simulink model "sat_dist_sim"  (R2023b)
settings: Solver=VariableStepAuto  StartTime=0.0  StopTime=10.0  RelTol=1e-3
values from neighbouring files (symbols this model uses):
  A = [0.49 0.49 0.49 0.49 0.49 0.49 0.49 0.49 0.49 0.49 0.49 0.49 0.49 0.49]    [disturbances_report.m]    (also in sat_dist.m = [6*1e-2; 6*1e-2; 6*1e-2; 6*1e-2; 4*1e-2; 4*1e-2; 12*1e-2; 12)
  a = 1 / ( (2/r) - (v^2 / mu) )    [car2par.m]    (also in disturbances_report.m = 6851.22197053)
  A0 = eye(3)    [sat_dist.m]
  e = norm(ee)    [car2par.m]    (also in disturbances_report.m = 0.00183012221618)
  e3 = [1; 0; 0]    [sat_dist.m]
  epsilon = astroConstants(8)    [sat_dist.m]
  H0 = sqrt(g01^2+g11^2+h11^2)*1e-9    [disturbances_report.m]    (also in sat_dist.m)
  I = diag([I1 I2 I3])    [sat_dist.m]
  i_matrix = [1 0 0;0 cos(i) sin(i); 0 -sin(i) cos(i)]    [sat_dist.m]
  Iinv = I\eye(3)    [sat_dist.m]
  incl = deg2rad(11.5)    [disturbances_report.m]    (also in sat_dist.m)
  jb = [0.01; 0.05; 0.01]    [disturbances_report.m]    (also in sat_dist.m)
  mu = 3.986 * 10^5    (= 398600)    [car2par.m]    (also in sat_dist.m = astroConstants(13))
  n = sqrt(mu/a^3)    [sat_dist.m]
  N = [1 0 0]'    [car2par.m]    (also in disturbances_report.m = [0 1 0; 0 -1 0; sqrt(2)/2 0 sqrt(2)/2; -sqrt(2)/2 0 sqrt(2)/; sat_dist.m = [1 0 0; 0 1 0; -1 0 0; 0 -1 0; 0 0 1; 0 0 -1; 1 0 0; -1 0 0;)
  ns = 2*pi / Ts    (= 1.99098639111e-07)    [sat_dist.m]
  omega0 = zeros(3,1)    [disturbances_report.m]    (also in sat_dist.m = [0; 0; n])
  omegaE = deg2rad(15)/3600    [disturbances_report.m]    (also in sat_dist.m)
  P = astroConstants(31)/(astroConstants(5)*10^3)    [disturbances_report.m]    (also in sat_dist.m = Fe/c)
  rf = 1e-2*[10 0 0; 0 10 0; -10 0 0; 0 -10 0; 0 0 15; 0 0 -15; 0 0 45; 0 0 45; 0 0 -45; 0 0 -45]    [sat_dist.m]
  rhod = 0.1*ones(10,1)    [sat_dist.m]
  rhos = 0.5*ones(10,1)    [sat_dist.m]
  rhos_ = ones(10,1)-rhos    [sat_dist.m]
  rs = -rr    [disturbances_report.m]    (also in sat_dist.m = astroConstants(2))
  Rt = astroConstants(23)    [disturbances_report.m]    (also in sat_dist.m)
  s0 = zeros(3,1)    [disturbances_report.m]    (also in sat_dist.m)
undefined symbols (not defined in the file or in its folder): phi0, psi0, theta0
libraries: matrix_library x13
settings Model: Creator=marcellopareschi  LastModifiedBy=marcellopareschi

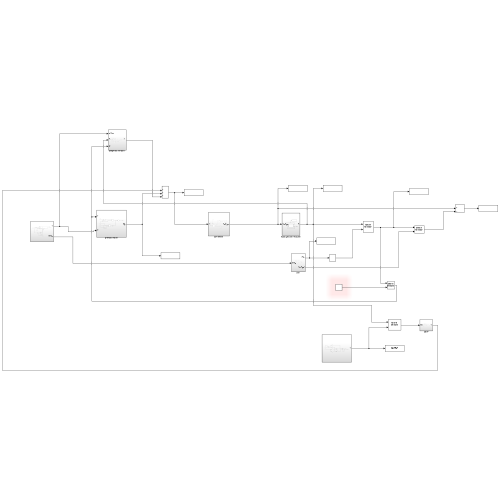
[thumbnail: Simulink's stored preview of the top-level diagram]
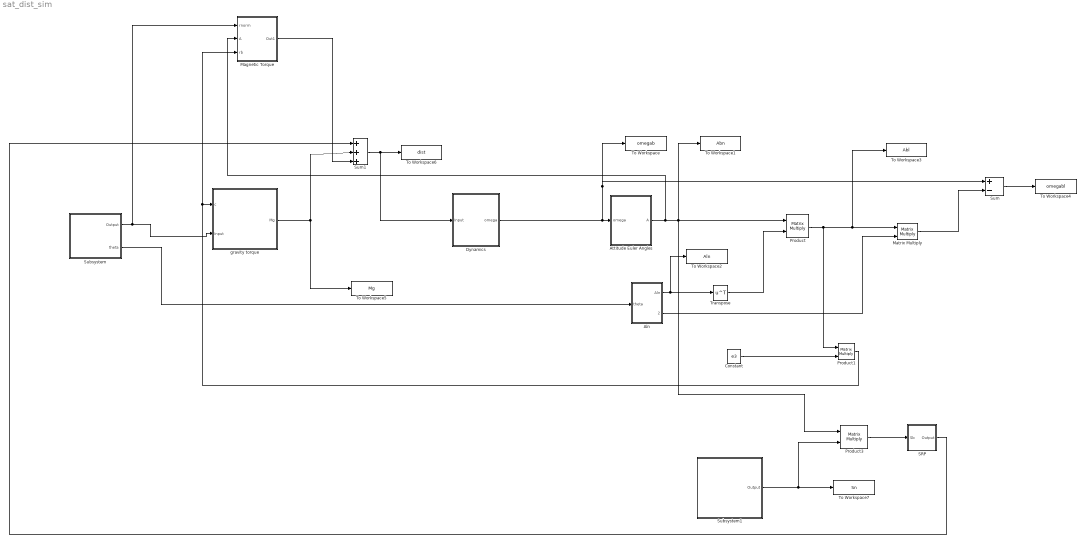
== system sat_dist_sim ==
  Aln : Subsystem
  Attitude Euler Angles : Subsystem
  Constant : Constant  Value=e3
  Dynamics : Subsystem
  "Magnetic Torque " : Subsystem
  Matrix Multiply : Product  Multiplication=Matrix(*)
  Product : Product  Multiplication=Matrix(*)
  Product1 : Product  Multiplication=Matrix(*)
  Product3 : Product  Multiplication=Matrix(*)
  SRP : Subsystem
  Subsystem : Subsystem
  Subsystem1 : Subsystem
  Sum : Sum  Inputs=|+-
  Sum1 : Sum  Inputs=|+++
  To Workspace : ToWorkspace  VariableName=omegab  SampleTime=-1
  To Workspace1 : ToWorkspace  VariableName=Abn  SampleTime=-1
  To Workspace2 : ToWorkspace  VariableName=Aln  SampleTime=-1
  To Workspace3 : ToWorkspace  VariableName=Abl  SampleTime=-1
  To Workspace4 : ToWorkspace  VariableName=omegabl  SampleTime=-1
  To Workspace5 : ToWorkspace  VariableName=Mg  SampleTime=-1
  To Workspace6 : ToWorkspace  VariableName=dist  SampleTime=-1
  To Workspace7 : ToWorkspace  VariableName=Sn  SampleTime=-1
  Transpose : Math  Operator=transpose
  gravity torque : Subsystem
  wires:
  Sum/1 -> To Workspace4/1
  Attitude Euler Angles/1(A) -> "Magnetic Torque "/2(A), Product3/1, To Workspace1/1, Product/1
  Product/1 -> To Workspace3/1, Matrix Multiply/1, Product1/1
  Aln/2(omegal) -> Matrix Multiply/2
  Transpose/1 -> Product/2
  Subsystem/2(theta) -> Aln/1(theta)
  Subsystem/1(Output) -> "Magnetic Torque "/1(rnorm), gravity torque/2(Input)
  Dynamics/1(omega) -> To Workspace/1, Sum/1, Attitude Euler Angles/1(omega)
  Aln/1(Aln) -> To Workspace2/1, Transpose/1
  Product3/1 -> SRP/1(Sb)
  Constant/1 -> Product1/2
  Product1/1 -> "Magnetic Torque "/3(rb), gravity torque/1(c)
  gravity torque/1(Mg) -> Sum1/2, To Workspace5/1
  Matrix Multiply/1 -> Sum/2
  SRP/1(Output) -> Sum1/1
  Subsystem1/1(Output) -> To Workspace7/1, Product3/2
  Sum1/1 -> Dynamics/1(Input), To Workspace6/1
  "Magnetic Torque "/1(Out1) -> Sum1/3

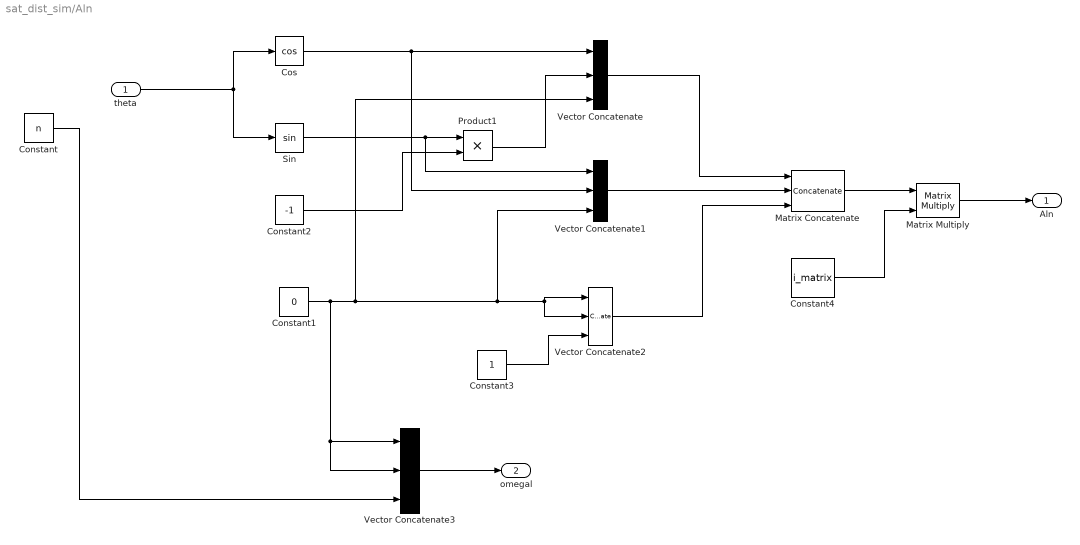
== system sat_dist_sim/Aln ==
  theta : Inport
  Constant : Constant  Value=n
  Constant1 : Constant  Value=0
  Constant2 : Constant  Value=-1
  Constant3 : Constant
  Constant4 : Constant  Value=i_matrix
  Cos : Trigonometry  Operator=cos
  Matrix Concatenate : Concatenate  NumInputs=3  Mode=Multidimensional array  ConcatenateDimension=2
  Matrix Multiply : Product  Multiplication=Matrix(*)
  Product1 : Product
  Sin : Trigonometry
  Vector Concatenate{,1..3} (4 alike) : Concatenate  NumInputs=3
  Aln : Outport
  omegal : Outport  Port=2
  wires:
  Constant/1 -> Vector Concatenate3/3
  Cos/1 -> Vector Concatenate1/2, Vector Concatenate/1
  Sin/1 -> Vector Concatenate1/1, Product1/1
  Constant2/1 -> Product1/2
  Product1/1 -> Vector Concatenate/2
  Constant1/1 -> Vector Concatenate3/1, Vector Concatenate3/2, Vector Concatenate/3, Vector Concatenate2/2, Vector Concatenate2/1, Vector Concatenate1/3
  Constant3/1 -> Vector Concatenate2/3
  Vector Concatenate/1 -> Matrix Concatenate/1
  Vector Concatenate1/1 -> Matrix Concatenate/2
  Vector Concatenate2/1 -> Matrix Concatenate/3
  Vector Concatenate3/1 -> omegal/1
  theta/1 -> Sin/1, Cos/1
  Matrix Concatenate/1 -> Matrix Multiply/1
  Constant4/1 -> Matrix Multiply/2
  Matrix Multiply/1 -> Aln/1

== system sat_dist_sim/Attitude Euler Angles ==
  omega : Inport
  Subsystem1 : Subsystem
  To Workspace : ToWorkspace  VariableName=angles  SampleTime=-1
  A : Outport
  wires:
  omega/1 -> Subsystem1/1(In1)
  Subsystem1/1(Angles) -> To Workspace/1, Subsystem1/2(Input)
  Subsystem1/2(A) -> Subsystem1/3(Input1), A/1

== system sat_dist_sim/Dynamics ==
  Input : Inport
  Constant : Constant  Value=I
  Constant1 : Constant  Value=Iinv
  Cross Product : matrix_library/Cross Product
  Integrator : Integrator  InitialCondition=omega0
  Product : Product  Multiplication=Matrix(*)
  Product1 : Product  Multiplication=Matrix(*)
  Scope : Scope
  Sum : Sum  Inputs=|++
  omega : Outport
  wires:
  Constant/1 -> Product/1
  Product1/1 -> Integrator/1
  Integrator/1 -> omega/1, Scope/1, Product/2, Cross Product/2
  Product/1 -> Cross Product/1
  Constant1/1 -> Product1/1
  Cross Product/1 -> Sum/1
  Sum/1 -> Product1/2
  Input/1 -> Sum/2

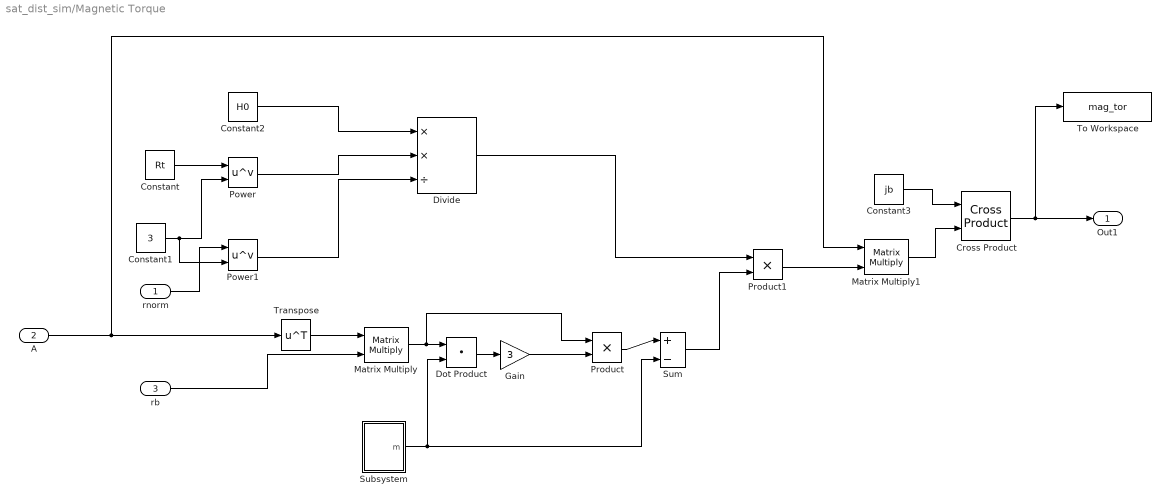
== system sat_dist_sim/Magnetic Torque  ==
  rnorm : Inport
  A : Inport  Port=2
  rb : Inport  Port=3
  Constant : Constant  Value=Rt
  Constant1 : Constant  Value=3
  Constant2 : Constant  Value=H0
  Constant3 : Constant  Value=jb
  Cross Product : matrix_library/Cross Product
  Divide : Product  Inputs=**/
  Dot Product : DotProduct  OutDataTypeStr=Inherit: Inherit via internal rule
  Gain : Gain  Gain=3
  Matrix Multiply : Product  Multiplication=Matrix(*)
  Matrix Multiply1 : Product  Multiplication=Matrix(*)
  Power : Math  Operator=pow
  Power1 : Math  Operator=pow
  Product : Product
  Product1 : Product
  Subsystem : Subsystem
  Sum : Sum  Inputs=|+-
  To Workspace : ToWorkspace  VariableName=mag_tor  SampleTime=-1
  Transpose : Math  Operator=transpose
  Out1 : Outport
  wires:
  A/1 -> Matrix Multiply1/1, Transpose/1
  Transpose/1 -> Matrix Multiply/1
  rb/1 -> Matrix Multiply/2
  Matrix Multiply/1 -> Product/1, Dot Product/1
  Subsystem/1(m) -> Sum/2, Dot Product/2
  Dot Product/1 -> Gain/1
  Gain/1 -> Product/2
  Product/1 -> Sum/1
  Constant/1 -> Power/1
  Constant1/1 -> Power1/2, Power/2
  rnorm/1 -> Power1/1
  Constant2/1 -> Divide/1
  Power/1 -> Divide/2
  Power1/1 -> Divide/3
  Divide/1 -> Product1/1
  Sum/1 -> Product1/2
  Product1/1 -> Matrix Multiply1/2
  Constant3/1 -> Cross Product/1
  Matrix Multiply1/1 -> Cross Product/2
  Cross Product/1 -> To Workspace/1, Out1/1

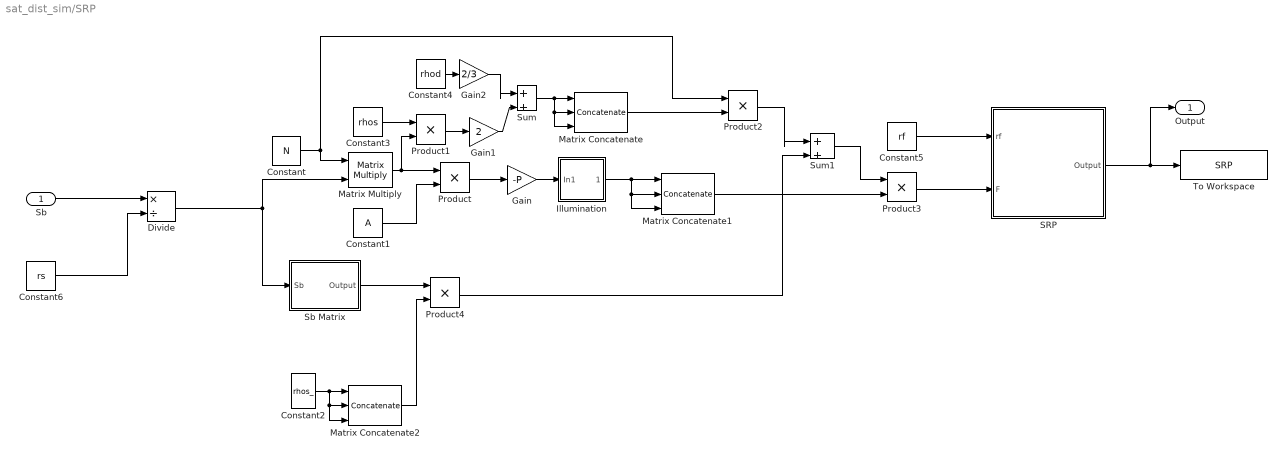
== system sat_dist_sim/SRP ==
  Sb : Inport
  Constant : Constant  Value=N
  Constant1 : Constant  Value=A
  Constant2 : Constant  Value=rhos_
  Constant3 : Constant  Value=rhos
  Constant4 : Constant  Value=rhod
  Constant5 : Constant  Value=rf
  Constant6 : Constant  Value=rs
  Divide : Product  Inputs=*/
  Gain : Gain  Gain=-P
  Gain1 : Gain  Gain=2
  Gain2 : Gain  Gain=2/3
  Illumination : Subsystem
  Matrix Concatenate : Concatenate  NumInputs=3  Mode=Multidimensional array  ConcatenateDimension=2
  Matrix Concatenate1 : Concatenate  NumInputs=3  Mode=Multidimensional array  ConcatenateDimension=2
  Matrix Concatenate2 : Concatenate  NumInputs=3  Mode=Multidimensional array  ConcatenateDimension=2
  Matrix Multiply : Product  Multiplication=Matrix(*)
  Product{,1..4} (5 alike) : Product
  SRP : Subsystem
  Sb Matrix : Subsystem
  Sum : Sum  Inputs=|++
  Sum1 : Sum  Inputs=|++
  To Workspace : ToWorkspace  VariableName=SRP  SampleTime=-1
  Output : Outport
  wires:
  Constant/1 -> Product2/1, Matrix Multiply/1
  Matrix Multiply/1 -> Product1/2, Product/1
  Constant1/1 -> Product/2
  Product/1 -> Gain/1
  Constant3/1 -> Product1/1
  Product1/1 -> Gain1/1
  Constant4/1 -> Gain2/1
  Gain2/1 -> Sum/1
  Gain1/1 -> Sum/2
  Sum/1 -> Matrix Concatenate/3, Matrix Concatenate/2, Matrix Concatenate/1
  Matrix Concatenate/1 -> Product2/2
  Gain/1 -> Illumination/1(In1)
  Product2/1 -> Sum1/1
  Matrix Concatenate1/1 -> Product3/2
  Sum1/1 -> Product3/1
  Constant5/1 -> SRP/1(rf)
  Product3/1 -> SRP/2(F)
  Constant2/1 -> Matrix Concatenate2/3, Matrix Concatenate2/2, Matrix Concatenate2/1
  Sb Matrix/1(Output) -> Product4/1
  Matrix Concatenate2/1 -> Product4/2
  Product4/1 -> Sum1/2
  Sb/1 -> Divide/1
  Constant6/1 -> Divide/2
  Divide/1 -> Sb Matrix/1(Sb), Matrix Multiply/2
  Illumination/1(Output) -> Matrix Concatenate1/3, Matrix Concatenate1/2, Matrix Concatenate1/1
  SRP/1(Output) -> To Workspace/1, Output/1

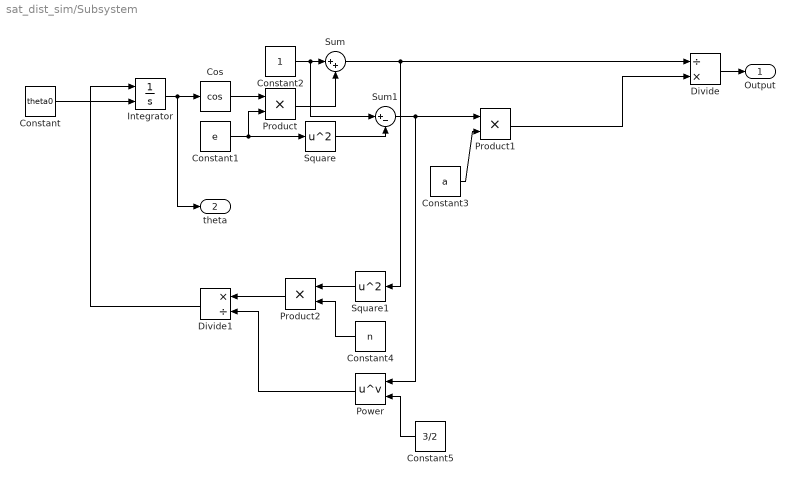
== system sat_dist_sim/Subsystem ==
  Constant : Constant  Value=theta0
  Constant1 : Constant  Value=e
  Constant2 : Constant
  Constant3 : Constant  Value=a
  Constant4 : Constant  Value=n
  Constant5 : Constant  Value=3/2
  Cos : Trigonometry  Operator=cos
  Divide : Product  Inputs=/*
  Divide1 : Product  Inputs=*/
  Integrator : Integrator  InitialConditionSource=external
  Power : Math  Operator=pow
  Product : Product
  Product1 : Product
  Product2 : Product
  Square : Math  Operator=square
  Square1 : Math  Operator=square
  Sum : Sum  Inputs=|++
  Sum1 : Sum  Inputs=|+-
  Output : Outport
  theta : Outport  Port=2
  wires:
  Constant/1 -> Integrator/2
  Integrator/1 -> theta/1, Cos/1
  Cos/1 -> Product/1
  Constant1/1 -> Square/1, Product/2
  Constant2/1 -> Sum1/1, Sum/1
  Product/1 -> Sum/2
  Square/1 -> Sum1/2
  Sum1/1 -> Power/1, Product1/1
  Constant3/1 -> Product1/2
  Product1/1 -> Divide/2
  Sum/1 -> Square1/1, Divide/1
  Square1/1 -> Product2/1
  Constant4/1 -> Product2/2
  Constant5/1 -> Power/2
  Product2/1 -> Divide1/1
  Power/1 -> Divide1/2
  Divide1/1 -> Integrator/1
  Divide/1 -> Output/1

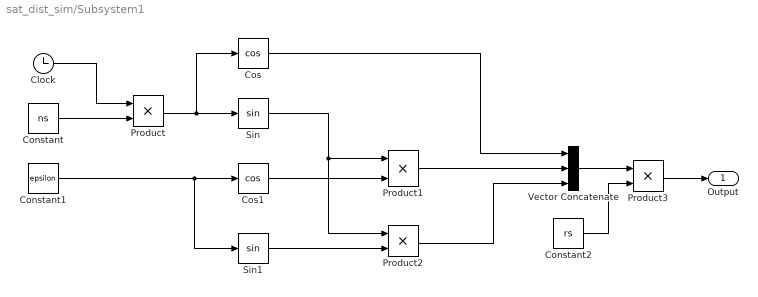
== system sat_dist_sim/Subsystem1 ==
  Clock : Clock
  Constant : Constant  Value=ns
  Constant1 : Constant  Value=epsilon
  Constant2 : Constant  Value=rs
  Cos : Trigonometry  Operator=cos
  Cos1 : Trigonometry  Operator=cos
  Product{,1..3} (4 alike) : Product
  Sin : Trigonometry
  Sin1 : Trigonometry
  Vector Concatenate : Concatenate  NumInputs=3
  Output : Outport
  wires:
  Constant/1 -> Product/2
  Clock/1 -> Product/1
  Product/1 -> Cos/1, Sin/1
  Constant1/1 -> Sin1/1, Cos1/1
  Sin/1 -> Product2/1, Product1/1
  Cos1/1 -> Product1/2
  Sin1/1 -> Product2/2
  Cos/1 -> Vector Concatenate/1
  Product1/1 -> Vector Concatenate/2
  Product2/1 -> Vector Concatenate/3
  Vector Concatenate/1 -> Product3/1
  Constant2/1 -> Product3/2
  Product3/1 -> Output/1

== system sat_dist_sim/gravity torque ==
  c : Inport
  Input : Inport  Port=2
  Constant : Constant  Value=mu
  Constant1 : Constant  Value=I
  Constant3 : Constant  Value=3
  Cross Product : matrix_library/Cross Product
  Divide : Product  Inputs=**/
  Gain : Gain  Gain=-1
  Matrix Multiply : Product  Multiplication=Matrix(*)
  Power : Math  Operator=pow
  Product : Product
  Mg : Outport
  wires:
  Constant1/1 -> Matrix Multiply/1
  c/1 -> Matrix Multiply/2, Cross Product/2
  Matrix Multiply/1 -> Cross Product/1
  Constant3/1 -> Power/2, Divide/2
  Power/1 -> Divide/3
  Constant/1 -> Divide/1
  Divide/1 -> Gain/1
  Gain/1 -> Product/2
  Cross Product/1 -> Product/1
  Product/1 -> Mg/1
  Input/1 -> Power/1

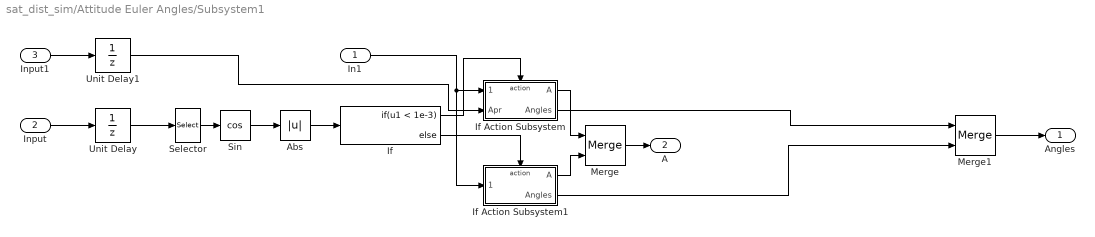
== system sat_dist_sim/Attitude Euler Angles/Subsystem1 ==
  In1 : Inport
  Input : Inport  Port=2
  Input1 : Inport  Port=3
  Abs : Abs  SaturateOnIntegerOverflow=off
  If : If  IfExpression=u1 < 1e-3
  If Action Subsystem : Subsystem  TreatAsAtomicUnit=on
  If Action Subsystem1 : Subsystem  TreatAsAtomicUnit=on
  Merge : Merge
  Merge1 : Merge
  Selector : Selector  InputPortWidth=3  IndexOptions=Index vector (dialog)  Indices=2  OutputSizes=1
  Sin : Trigonometry  Operator=cos
  Unit Delay : UnitDelay  InitialCondition=s0  SampleTime=-1  HasFrameUpgradeWarning=on
  Unit Delay1 : UnitDelay  InitialCondition=A0  SampleTime=-1  HasFrameUpgradeWarning=on
  Angles : Outport
  A : Outport  Port=2
  wires:
  Input/1 -> Unit Delay/1
  Unit Delay/1 -> Selector/1
  Sin/1 -> Abs/1
  Abs/1 -> If/1
  If/1 -> If Action Subsystem/Action
  If/2 -> If Action Subsystem1/Action
  If Action Subsystem1/1(A) -> Merge/2
  If Action Subsystem/1(A) -> Merge/1
  In1/1 -> If Action Subsystem1/1(omega), If Action Subsystem/1(omega)
  Selector/1 -> Sin/1
  If Action Subsystem1/2(Angles) -> Merge1/2
  If Action Subsystem/2(Angles) -> Merge1/1
  Merge1/1 -> Angles/1
  Merge/1 -> A/1
  Input1/1 -> Unit Delay1/1
  Unit Delay1/1 -> If Action Subsystem/2(Apr)

== system sat_dist_sim/Magnetic Torque /Subsystem ==
  Clock : Clock
  Constant : Constant  Value=incl
  Constant1 : Constant  Value=omegaE
  Cos : Trigonometry  Operator=cos
  Cos1 : Trigonometry  Operator=cos
  Product : Product
  Product1 : Product
  Product2 : Product
  Sin : Trigonometry
  Sin1 : Trigonometry
  Vector Concatenate : Concatenate  NumInputs=3
  m : Outport
  wires:
  Constant/1 -> Cos/1, Sin/1
  Clock/1 -> Product/1
  Constant1/1 -> Product/2
  Product/1 -> Sin1/1, Cos1/1
  Cos1/1 -> Product1/1
  Sin/1 -> Product2/2, Product1/2
  Sin1/1 -> Product2/1
  Product1/1 -> Vector Concatenate/1
  Product2/1 -> Vector Concatenate/2
  Cos/1 -> Vector Concatenate/3
  Vector Concatenate/1 -> m/1

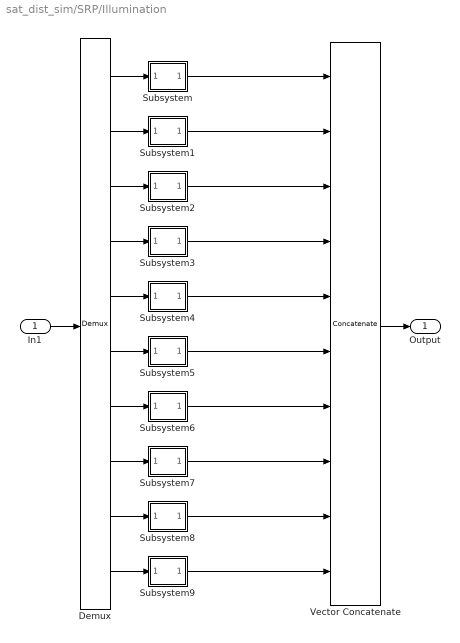
== system sat_dist_sim/SRP/Illumination ==
  In1 : Inport
  Demux : Demux  Outputs=10
  Subsystem : Subsystem
  Subsystem1 : Subsystem
  Subsystem2 : Subsystem
  Subsystem3 : Subsystem
  Subsystem4 : Subsystem
  Subsystem5 : Subsystem
  Subsystem6 : Subsystem
  Subsystem7 : Subsystem
  Subsystem8 : Subsystem
  Subsystem9 : Subsystem
  Vector Concatenate : Concatenate  NumInputs=10
  Output : Outport
  wires:
  In1/1 -> Demux/1
  Demux/1 -> Subsystem/1(In1)
  Demux/2 -> Subsystem1/1(In1)
  Demux/3 -> Subsystem2/1(In1)
  Demux/4 -> Subsystem3/1(In1)
  Demux/5 -> Subsystem4/1(In1)
  Demux/6 -> Subsystem5/1(In1)
  Demux/7 -> Subsystem6/1(In1)
  Demux/8 -> Subsystem7/1(In1)
  Demux/9 -> Subsystem8/1(In1)
  Demux/10 -> Subsystem9/1(In1)
  Subsystem/1(Output) -> Vector Concatenate/1
  Subsystem1/1(Output) -> Vector Concatenate/2
  Subsystem2/1(Output) -> Vector Concatenate/3
  Subsystem3/1(Output) -> Vector Concatenate/4
  Subsystem4/1(Output) -> Vector Concatenate/5
  Subsystem5/1(Output) -> Vector Concatenate/6
  Subsystem6/1(Output) -> Vector Concatenate/7
  Subsystem7/1(Output) -> Vector Concatenate/8
  Subsystem8/1(Output) -> Vector Concatenate/9
  Subsystem9/1(Output) -> Vector Concatenate/10
  Vector Concatenate/1 -> Output/1

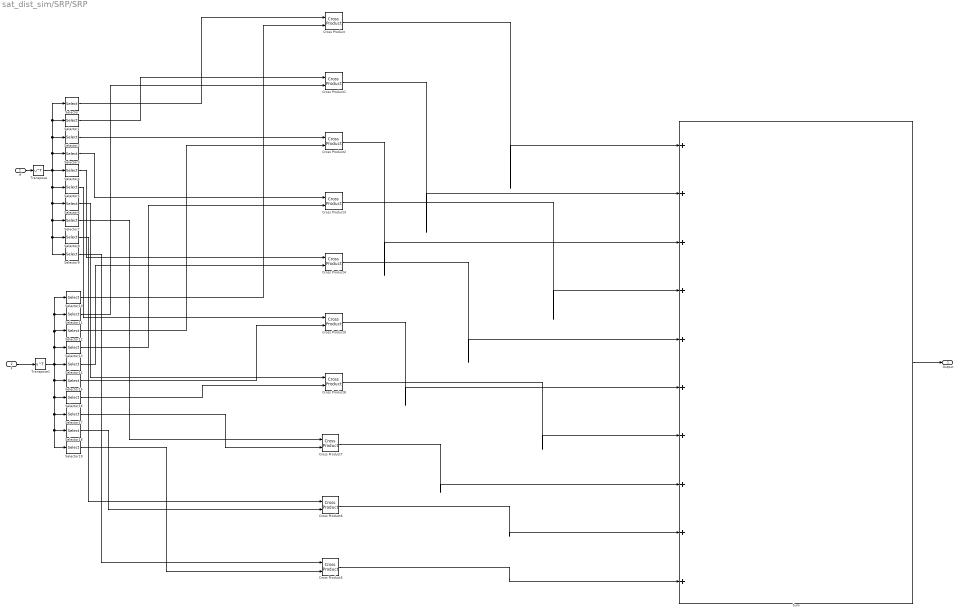
== system sat_dist_sim/SRP/SRP ==
  rf : Inport
  F : Inport  Port=2
  Cross Product{,1..9} (10 alike) : matrix_library/Cross Product
  Selector : Selector  NumberOfDimensions=2  InputPortWidth=3  IndexOptions=Index vector (dialog),Index vector (dialog)  Indices=[1 2 3],1  OutputSizes=1,1
  Selector1 : Selector  NumberOfDimensions=2  InputPortWidth=3  IndexOptions=Index vector (dialog),Index vector (dialog)  Indices=[1 2 3],2  OutputSizes=1,1
  Selector10 : Selector  NumberOfDimensions=2  InputPortWidth=3  IndexOptions=Index vector (dialog),Index vector (dialog)  Indices=[1 2 3],1  OutputSizes=1,1
  Selector11 : Selector  NumberOfDimensions=2  InputPortWidth=3  IndexOptions=Index vector (dialog),Index vector (dialog)  Indices=[1 2 3],2  OutputSizes=1,1
  Selector12 : Selector  NumberOfDimensions=2  InputPortWidth=3  IndexOptions=Index vector (dialog),Index vector (dialog)  Indices=[1 2 3],3  OutputSizes=1,1
  Selector13 : Selector  NumberOfDimensions=2  InputPortWidth=3  IndexOptions=Index vector (dialog),Index vector (dialog)  Indices=[1 2 3],4  OutputSizes=1,1
  Selector14 : Selector  NumberOfDimensions=2  InputPortWidth=3  IndexOptions=Index vector (dialog),Index vector (dialog)  Indices=[1 2 3],5  OutputSizes=1,1
  Selector15 : Selector  NumberOfDimensions=2  InputPortWidth=3  IndexOptions=Index vector (dialog),Index vector (dialog)  Indices=[1 2 3],6  OutputSizes=1,1
  Selector16 : Selector  NumberOfDimensions=2  InputPortWidth=3  IndexOptions=Index vector (dialog),Index vector (dialog)  Indices=[1 2 3],7  OutputSizes=1,1
  Selector17 : Selector  NumberOfDimensions=2  InputPortWidth=3  IndexOptions=Index vector (dialog),Index vector (dialog)  Indices=[1 2 3],8  OutputSizes=1,1
  Selector18 : Selector  NumberOfDimensions=2  InputPortWidth=3  IndexOptions=Index vector (dialog),Index vector (dialog)  Indices=[1 2 3],9  OutputSizes=1,1
  Selector19 : Selector  NumberOfDimensions=2  InputPortWidth=3  IndexOptions=Index vector (dialog),Index vector (dialog)  Indices=[1 2 3],10  OutputSizes=1,1
  Selector2 : Selector  NumberOfDimensions=2  InputPortWidth=3  IndexOptions=Index vector (dialog),Index vector (dialog)  Indices=[1 2 3],3  OutputSizes=1,1
  Selector3 : Selector  NumberOfDimensions=2  InputPortWidth=3  IndexOptions=Index vector (dialog),Index vector (dialog)  Indices=[1 2 3],4  OutputSizes=1,1
  Selector4 : Selector  NumberOfDimensions=2  InputPortWidth=3  IndexOptions=Index vector (dialog),Index vector (dialog)  Indices=[1 2 3],5  OutputSizes=1,1
  Selector5 : Selector  NumberOfDimensions=2  InputPortWidth=3  IndexOptions=Index vector (dialog),Index vector (dialog)  Indices=[1 2 3],6  OutputSizes=1,1
  Selector6 : Selector  NumberOfDimensions=2  InputPortWidth=3  IndexOptions=Index vector (dialog),Index vector (dialog)  Indices=[1 2 3],7  OutputSizes=1,1
  Selector7 : Selector  NumberOfDimensions=2  InputPortWidth=3  IndexOptions=Index vector (dialog),Index vector (dialog)  Indices=[1 2 3],8  OutputSizes=1,1
  Selector8 : Selector  NumberOfDimensions=2  InputPortWidth=3  IndexOptions=Index vector (dialog),Index vector (dialog)  Indices=[1 2 3],9  OutputSizes=1,1
  Selector9 : Selector  NumberOfDimensions=2  InputPortWidth=3  IndexOptions=Index vector (dialog),Index vector (dialog)  Indices=[1 2 3],10  OutputSizes=1,1
  Sum : Sum  Inputs=|++++++++++
  Transpose : Math  Operator=transpose
  Transpose1 : Math  Operator=transpose
  Output : Outport
  wires:
  rf/1 -> Transpose/1
  Transpose/1 -> Selector6/1, Selector9/1, Selector8/1, Selector7/1, Selector5/1, Selector3/1, Selector2/1, Selector1/1, Selector/1, Selector4/1
  Transpose1/1 -> Selector16/1, Selector19/1, Selector18/1, Selector17/1, Selector15/1, Selector13/1, Selector12/1, Selector11/1, Selector10/1, Selector14/1
  F/1 -> Transpose1/1
  Selector/1 -> Cross Product/1
  Selector10/1 -> Cross Product/2
  Selector1/1 -> Cross Product1/1
  Selector11/1 -> Cross Product1/2
  Selector2/1 -> Cross Product2/1
  Selector12/1 -> Cross Product2/2
  Selector3/1 -> Cross Product3/1
  Selector13/1 -> Cross Product3/2
  Selector4/1 -> Cross Product4/1
  Selector14/1 -> Cross Product4/2
  Selector5/1 -> Cross Product9/1
  Selector15/1 -> Cross Product9/2
  Selector6/1 -> Cross Product8/1
  Selector16/1 -> Cross Product8/2
  Selector7/1 -> Cross Product7/1
  Selector17/1 -> Cross Product7/2
  Selector8/1 -> Cross Product6/1
  Selector18/1 -> Cross Product6/2
  Selector9/1 -> Cross Product5/1
  Selector19/1 -> Cross Product5/2
  Cross Product/1 -> Sum/1
  Cross Product1/1 -> Sum/2
  Cross Product2/1 -> Sum/3
  Cross Product3/1 -> Sum/4
  Cross Product4/1 -> Sum/5
  Cross Product9/1 -> Sum/6
  Cross Product8/1 -> Sum/7
  Cross Product7/1 -> Sum/8
  Cross Product6/1 -> Sum/9
  Cross Product5/1 -> Sum/10
  Sum/1 -> Output/1

== system sat_dist_sim/SRP/Sb Matrix ==
  Sb : Inport
  Matrix Concatenate : Concatenate  NumInputs=10  Mode=Multidimensional array
  Transpose : Math  Operator=transpose
  Output : Outport
  wires:
  Sb/1 -> Transpose/1
  Transpose/1 -> Matrix Concatenate/4, Matrix Concatenate/5, Matrix Concatenate/6, Matrix Concatenate/7, Matrix Concatenate/8, Matrix Concatenate/9, Matrix Concatenate/10, Matrix Concatenate/1, Matrix Concatenate/2, Matrix Concatenate/3
  Matrix Concatenate/1 -> Output/1

== system sat_dist_sim/Attitude Euler Angles/Subsystem1/If Action Subsystem ==
  omega : Inport
  Apr : Inport  Port=2
  Action Port : ActionPort  ActionPortLabel=if(u1 < 1e-3)
  "Kin 313 " : Subsystem
  conversion 313 312 : Subsystem
  conversion from 312 to 313 : Subsystem
  A : Outport
  Angles : Outport  Port=2
  wires:
  Apr/1 -> conversion from 312 to 313/1(Apr)
  conversion from 312 to 313/1(Angles) -> "Kin 313 "/2(Angles)
  omega/1 -> "Kin 313 "/1(omega)
  "Kin 313 "/1(A) -> conversion 313 312/1(A), A/1
  conversion 313 312/1(Angles) -> Angles/1

== system sat_dist_sim/Attitude Euler Angles/Subsystem1/If Action Subsystem1 ==
  omega : Inport
  Action Port : ActionPort  ActionPortLabel=else
  Kin 312 : Subsystem
  A : Outport
  Angles : Outport  Port=2
  wires:
  Kin 312/1(A) -> A/1
  omega/1 -> Kin 312/1(omega)
  Kin 312/2(Angles) -> Angles/1

== system sat_dist_sim/SRP/Illumination/Subsystem ==
  In1 : Inport
  If : If
  If Action Subsystem : Subsystem  TreatAsAtomicUnit=on
  If Action Subsystem1 : Subsystem  TreatAsAtomicUnit=on
  Merge : Merge
  Output : Outport
  wires:
  In1/1 -> If Action Subsystem1/1(In1), If Action Subsystem/1(In1), If/1
  If/1 -> If Action Subsystem/Action
  If/2 -> If Action Subsystem1/Action
  If Action Subsystem/1(Out1) -> Merge/1
  If Action Subsystem1/1(Out1) -> Merge/2
  Merge/1 -> Output/1

== system sat_dist_sim/SRP/Illumination/Subsystem1 ==
  In1 : Inport
  If : If
  If Action Subsystem : Subsystem  TreatAsAtomicUnit=on
  If Action Subsystem1 : Subsystem  TreatAsAtomicUnit=on
  Merge : Merge
  Output : Outport
  wires:
  In1/1 -> If Action Subsystem1/1(In1), If Action Subsystem/1(In1), If/1
  If/1 -> If Action Subsystem/Action
  If/2 -> If Action Subsystem1/Action
  If Action Subsystem/1(Out1) -> Merge/1
  If Action Subsystem1/1(Out1) -> Merge/2
  Merge/1 -> Output/1

== system sat_dist_sim/SRP/Illumination/Subsystem2 ==
  In1 : Inport
  If : If
  If Action Subsystem : Subsystem  TreatAsAtomicUnit=on
  If Action Subsystem1 : Subsystem  TreatAsAtomicUnit=on
  Merge : Merge
  Output : Outport
  wires:
  In1/1 -> If Action Subsystem1/1(In1), If Action Subsystem/1(In1), If/1
  If/1 -> If Action Subsystem/Action
  If/2 -> If Action Subsystem1/Action
  If Action Subsystem/1(Out1) -> Merge/1
  If Action Subsystem1/1(Out1) -> Merge/2
  Merge/1 -> Output/1

== system sat_dist_sim/SRP/Illumination/Subsystem3 ==
  In1 : Inport
  If : If
  If Action Subsystem : Subsystem  TreatAsAtomicUnit=on
  If Action Subsystem1 : Subsystem  TreatAsAtomicUnit=on
  Merge : Merge
  Output : Outport
  wires:
  In1/1 -> If Action Subsystem1/1(In1), If Action Subsystem/1(In1), If/1
  If/1 -> If Action Subsystem/Action
  If/2 -> If Action Subsystem1/Action
  If Action Subsystem/1(Out1) -> Merge/1
  If Action Subsystem1/1(Out1) -> Merge/2
  Merge/1 -> Output/1

== system sat_dist_sim/SRP/Illumination/Subsystem4 ==
  In1 : Inport
  If : If
  If Action Subsystem : Subsystem  TreatAsAtomicUnit=on
  If Action Subsystem1 : Subsystem  TreatAsAtomicUnit=on
  Merge : Merge
  Output : Outport
  wires:
  In1/1 -> If Action Subsystem1/1(In1), If Action Subsystem/1(In1), If/1
  If/1 -> If Action Subsystem/Action
  If/2 -> If Action Subsystem1/Action
  If Action Subsystem/1(Out1) -> Merge/1
  If Action Subsystem1/1(Out1) -> Merge/2
  Merge/1 -> Output/1

== system sat_dist_sim/SRP/Illumination/Subsystem5 ==
  In1 : Inport
  If : If
  If Action Subsystem : Subsystem  TreatAsAtomicUnit=on
  If Action Subsystem1 : Subsystem  TreatAsAtomicUnit=on
  Merge : Merge
  Output : Outport
  wires:
  In1/1 -> If Action Subsystem1/1(In1), If Action Subsystem/1(In1), If/1
  If/1 -> If Action Subsystem/Action
  If/2 -> If Action Subsystem1/Action
  If Action Subsystem/1(Out1) -> Merge/1
  If Action Subsystem1/1(Out1) -> Merge/2
  Merge/1 -> Output/1

== system sat_dist_sim/SRP/Illumination/Subsystem6 ==
  In1 : Inport
  If : If
  If Action Subsystem : Subsystem  TreatAsAtomicUnit=on
  If Action Subsystem1 : Subsystem  TreatAsAtomicUnit=on
  Merge : Merge
  Output : Outport
  wires:
  In1/1 -> If Action Subsystem1/1(In1), If Action Subsystem/1(In1), If/1
  If/1 -> If Action Subsystem/Action
  If/2 -> If Action Subsystem1/Action
  If Action Subsystem/1(Out1) -> Merge/1
  If Action Subsystem1/1(Out1) -> Merge/2
  Merge/1 -> Output/1

== system sat_dist_sim/SRP/Illumination/Subsystem7 ==
  In1 : Inport
  If : If
  If Action Subsystem : Subsystem  TreatAsAtomicUnit=on
  If Action Subsystem1 : Subsystem  TreatAsAtomicUnit=on
  Merge : Merge
  Output : Outport
  wires:
  In1/1 -> If Action Subsystem1/1(In1), If Action Subsystem/1(In1), If/1
  If/1 -> If Action Subsystem/Action
  If/2 -> If Action Subsystem1/Action
  If Action Subsystem/1(Out1) -> Merge/1
  If Action Subsystem1/1(Out1) -> Merge/2
  Merge/1 -> Output/1

== system sat_dist_sim/SRP/Illumination/Subsystem8 ==
  In1 : Inport
  If : If
  If Action Subsystem : Subsystem  TreatAsAtomicUnit=on
  If Action Subsystem1 : Subsystem  TreatAsAtomicUnit=on
  Merge : Merge
  Output : Outport
  wires:
  In1/1 -> If Action Subsystem1/1(In1), If Action Subsystem/1(In1), If/1
  If/1 -> If Action Subsystem/Action
  If/2 -> If Action Subsystem1/Action
  If Action Subsystem/1(Out1) -> Merge/1
  If Action Subsystem1/1(Out1) -> Merge/2
  Merge/1 -> Output/1

== system sat_dist_sim/SRP/Illumination/Subsystem9 ==
  In1 : Inport
  If : If
  If Action Subsystem : Subsystem  TreatAsAtomicUnit=on
  If Action Subsystem1 : Subsystem  TreatAsAtomicUnit=on
  Merge : Merge
  Output : Outport
  wires:
  In1/1 -> If Action Subsystem1/1(In1), If Action Subsystem/1(In1), If/1
  If/1 -> If Action Subsystem/Action
  If/2 -> If Action Subsystem1/Action
  If Action Subsystem/1(Out1) -> Merge/1
  If Action Subsystem1/1(Out1) -> Merge/2
  Merge/1 -> Output/1

== system sat_dist_sim/Attitude Euler Angles/Subsystem1/If Action Subsystem/Kin 313  ==
  omega : Inport
  Angles : Inport  Port=2
  Subsystem : Subsystem
  Subsystem1 : Subsystem
  A : Outport
  wires:
  omega/1 -> Subsystem/1(omega)
  Subsystem/1(Phi) -> Subsystem1/1(Phi)
  Subsystem/2(Theta) -> Subsystem1/2(Theta)
  Subsystem/3(Psi) -> Subsystem1/3(Psi)
  Angles/1 -> Subsystem/2(Input)
  Subsystem1/1(A) -> A/1

== system sat_dist_sim/Attitude Euler Angles/Subsystem1/If Action Subsystem/conversion 313 312 ==
  A : Inport
  Asin : Trigonometry  Operator=asin
  Atan1 : Trigonometry  Operator=atan2
  Atan2 : Trigonometry  Operator=atan2
  Gain : Gain  Gain=-1
  Gain1 : Gain
  Selector : Selector  NumberOfDimensions=2  InputPortWidth=3  IndexOptions=Index vector (dialog),Index vector (dialog)  Indices=1,3  OutputSizes=1,1
  Selector1 : Selector  NumberOfDimensions=2  InputPortWidth=3  IndexOptions=Index vector (dialog),Index vector (dialog)  Indices=3,3  OutputSizes=1,1
  Selector2 : Selector  NumberOfDimensions=2  InputPortWidth=3  IndexOptions=Index vector (dialog),Index vector (dialog)  Indices=2,3  OutputSizes=1,1
  Selector3 : Selector  NumberOfDimensions=2  InputPortWidth=3  IndexOptions=Index vector (dialog),Index vector (dialog)  Indices=2,1  OutputSizes=1,1
  Selector4 : Selector  NumberOfDimensions=2  InputPortWidth=3  IndexOptions=Index vector (dialog),Index vector (dialog)  Indices=2,2  OutputSizes=1,1
  Vector Concatenate : Concatenate  NumInputs=3
  Angles : Outport
  wires:
  Selector/1 -> Gain/1
  Gain/1 -> Atan2/1
  Selector1/1 -> Atan2/2
  A/1 -> Selector1/1, Selector/1, Selector4/1, Selector3/1, Selector2/1
  Selector2/1 -> Asin/1
  Selector3/1 -> Gain1/1
  Gain1/1 -> Atan1/1
  Selector4/1 -> Atan1/2
  Asin/1 -> Vector Concatenate/2
  Atan2/1 -> Vector Concatenate/1
  Atan1/1 -> Vector Concatenate/3
  Vector Concatenate/1 -> Angles/1

== system sat_dist_sim/Attitude Euler Angles/Subsystem1/If Action Subsystem/conversion from 312 to 313 ==
  Apr : Inport
  Acos : Trigonometry  Operator=acos
  Atan1 : Trigonometry  Operator=atan2
  Atan2 : Trigonometry  Operator=atan2
  Gain : Gain  Gain=-1
  Selector : Selector  NumberOfDimensions=2  InputPortWidth=3  IndexOptions=Index vector (dialog),Index vector (dialog)  Indices=1,3  OutputSizes=1,1
  Selector1 : Selector  NumberOfDimensions=2  InputPortWidth=3  IndexOptions=Index vector (dialog),Index vector (dialog)  Indices=2,3  OutputSizes=1,1
  Selector2 : Selector  NumberOfDimensions=2  InputPortWidth=3  IndexOptions=Index vector (dialog),Index vector (dialog)  Indices=3,3  OutputSizes=1,1
  Selector3 : Selector  NumberOfDimensions=2  InputPortWidth=3  IndexOptions=Index vector (dialog),Index vector (dialog)  Indices=3,2  OutputSizes=1,1
  Selector4 : Selector  NumberOfDimensions=2  InputPortWidth=3  IndexOptions=Index vector (dialog),Index vector (dialog)  Indices=3,1  OutputSizes=1,1
  Vector Concatenate : Concatenate  NumInputs=3
  Angles : Outport
  wires:
  Apr/1 -> Selector/1, Selector1/1, Selector3/1, Selector4/1, Selector2/1
  Selector/1 -> Atan2/1
  Selector1/1 -> Atan2/2
  Selector2/1 -> Acos/1
  Selector4/1 -> Atan1/1
  Acos/1 -> Vector Concatenate/2
  Atan2/1 -> Vector Concatenate/1
  Atan1/1 -> Vector Concatenate/3
  Vector Concatenate/1 -> Angles/1
  Selector3/1 -> Gain/1
  Gain/1 -> Atan1/2

== system sat_dist_sim/Attitude Euler Angles/Subsystem1/If Action Subsystem1/Kin 312 ==
  omega : Inport
  Euler Angles : Subsystem
  Subsystem : Subsystem
  Vector Concatenate : Concatenate  NumInputs=3
  A : Outport
  Angles : Outport  Port=2
  wires:
  Euler Angles/1(Phi) -> Subsystem/1(phi), Vector Concatenate/3
  Euler Angles/2(Theta) -> Subsystem/2(theta), Vector Concatenate/2
  omega/1 -> Euler Angles/1(omega)
  Euler Angles/3(Psi) -> Subsystem/3(psi), Vector Concatenate/1
  Vector Concatenate/1 -> Angles/1
  Subsystem/1(A) -> A/1

== system sat_dist_sim/SRP/Illumination/Subsystem/If Action Subsystem ==
  In1 : Inport
  Action Port : ActionPort  ActionPortLabel=if(u1 > 0)
  Constant : Constant  Value=0
  Product : Product
  Out1 : Outport
  wires:
  In1/1 -> Product/1
  Constant/1 -> Product/2
  Product/1 -> Out1/1

== system sat_dist_sim/SRP/Illumination/Subsystem/If Action Subsystem1 ==
  In1 : Inport
  Action Port : ActionPort  ActionPortLabel=else
  Out1 : Outport
  wires:
  In1/1 -> Out1/1

== system sat_dist_sim/SRP/Illumination/Subsystem1/If Action Subsystem ==
  In1 : Inport
  Action Port : ActionPort  ActionPortLabel=if(u1 > 0)
  Constant : Constant  Value=0
  Product : Product
  Out1 : Outport
  wires:
  In1/1 -> Product/1
  Constant/1 -> Product/2
  Product/1 -> Out1/1

== system sat_dist_sim/SRP/Illumination/Subsystem1/If Action Subsystem1 ==
  In1 : Inport
  Action Port : ActionPort  ActionPortLabel=else
  Out1 : Outport
  wires:
  In1/1 -> Out1/1

== system sat_dist_sim/SRP/Illumination/Subsystem2/If Action Subsystem ==
  In1 : Inport
  Action Port : ActionPort  ActionPortLabel=if(u1 > 0)
  Constant : Constant  Value=0
  Product : Product
  Out1 : Outport
  wires:
  In1/1 -> Product/1
  Constant/1 -> Product/2
  Product/1 -> Out1/1

== system sat_dist_sim/SRP/Illumination/Subsystem2/If Action Subsystem1 ==
  In1 : Inport
  Action Port : ActionPort  ActionPortLabel=else
  Out1 : Outport
  wires:
  In1/1 -> Out1/1

== system sat_dist_sim/SRP/Illumination/Subsystem3/If Action Subsystem ==
  In1 : Inport
  Action Port : ActionPort  ActionPortLabel=if(u1 > 0)
  Constant : Constant  Value=0
  Product : Product
  Out1 : Outport
  wires:
  In1/1 -> Product/1
  Constant/1 -> Product/2
  Product/1 -> Out1/1

== system sat_dist_sim/SRP/Illumination/Subsystem3/If Action Subsystem1 ==
  In1 : Inport
  Action Port : ActionPort  ActionPortLabel=else
  Out1 : Outport
  wires:
  In1/1 -> Out1/1

== system sat_dist_sim/SRP/Illumination/Subsystem4/If Action Subsystem ==
  In1 : Inport
  Action Port : ActionPort  ActionPortLabel=if(u1 > 0)
  Constant : Constant  Value=0
  Product : Product
  Out1 : Outport
  wires:
  In1/1 -> Product/1
  Constant/1 -> Product/2
  Product/1 -> Out1/1

== system sat_dist_sim/SRP/Illumination/Subsystem4/If Action Subsystem1 ==
  In1 : Inport
  Action Port : ActionPort  ActionPortLabel=else
  Out1 : Outport
  wires:
  In1/1 -> Out1/1

== system sat_dist_sim/SRP/Illumination/Subsystem5/If Action Subsystem ==
  In1 : Inport
  Action Port : ActionPort  ActionPortLabel=if(u1 > 0)
  Constant : Constant  Value=0
  Product : Product
  Out1 : Outport
  wires:
  In1/1 -> Product/1
  Constant/1 -> Product/2
  Product/1 -> Out1/1

== system sat_dist_sim/SRP/Illumination/Subsystem5/If Action Subsystem1 ==
  In1 : Inport
  Action Port : ActionPort  ActionPortLabel=else
  Out1 : Outport
  wires:
  In1/1 -> Out1/1

== system sat_dist_sim/SRP/Illumination/Subsystem6/If Action Subsystem ==
  In1 : Inport
  Action Port : ActionPort  ActionPortLabel=if(u1 > 0)
  Constant : Constant  Value=0
  Product : Product
  Out1 : Outport
  wires:
  In1/1 -> Product/1
  Constant/1 -> Product/2
  Product/1 -> Out1/1

== system sat_dist_sim/SRP/Illumination/Subsystem6/If Action Subsystem1 ==
  In1 : Inport
  Action Port : ActionPort  ActionPortLabel=else
  Out1 : Outport
  wires:
  In1/1 -> Out1/1

== system sat_dist_sim/SRP/Illumination/Subsystem7/If Action Subsystem ==
  In1 : Inport
  Action Port : ActionPort  ActionPortLabel=if(u1 > 0)
  Constant : Constant  Value=0
  Product : Product
  Out1 : Outport
  wires:
  In1/1 -> Product/1
  Constant/1 -> Product/2
  Product/1 -> Out1/1

== system sat_dist_sim/SRP/Illumination/Subsystem7/If Action Subsystem1 ==
  In1 : Inport
  Action Port : ActionPort  ActionPortLabel=else
  Out1 : Outport
  wires:
  In1/1 -> Out1/1

== system sat_dist_sim/SRP/Illumination/Subsystem8/If Action Subsystem ==
  In1 : Inport
  Action Port : ActionPort  ActionPortLabel=if(u1 > 0)
  Constant : Constant  Value=0
  Product : Product
  Out1 : Outport
  wires:
  In1/1 -> Product/1
  Constant/1 -> Product/2
  Product/1 -> Out1/1

== system sat_dist_sim/SRP/Illumination/Subsystem8/If Action Subsystem1 ==
  In1 : Inport
  Action Port : ActionPort  ActionPortLabel=else
  Out1 : Outport
  wires:
  In1/1 -> Out1/1

== system sat_dist_sim/SRP/Illumination/Subsystem9/If Action Subsystem ==
  In1 : Inport
  Action Port : ActionPort  ActionPortLabel=if(u1 > 0)
  Constant : Constant  Value=0
  Product : Product
  Out1 : Outport
  wires:
  In1/1 -> Product/1
  Constant/1 -> Product/2
  Product/1 -> Out1/1

== system sat_dist_sim/SRP/Illumination/Subsystem9/If Action Subsystem1 ==
  In1 : Inport
  Action Port : ActionPort  ActionPortLabel=else
  Out1 : Outport
  wires:
  In1/1 -> Out1/1

== system sat_dist_sim/Attitude Euler Angles/Subsystem1/If Action Subsystem/Kin 313 /Subsystem ==
  omega : Inport
  Input : Inport  Port=2
  Demux : Demux  Outputs=3
  phi : Subsystem
  psi : Subsystem
  theta : Subsystem
  Phi : Outport
  Theta : Outport  Port=2
  Psi : Outport  Port=3
  wires:
  phi/1(phi) -> Phi/1
  omega/1 -> psi/1(omega), phi/1(omega), theta/1(omega)
  psi/1(psi) -> theta/2(psi), phi/2(theta), psi/2(Psi), Psi/1
  theta/1(theta) -> Theta/1, psi/3(theta), phi/3(psi)
  Input/1 -> Demux/1
  Demux/1 -> psi/4(Input)
  Demux/2 -> theta/3(Input)
  Demux/3 -> phi/4(Input)

== system sat_dist_sim/Attitude Euler Angles/Subsystem1/If Action Subsystem/Kin 313 /Subsystem1 ==
  Phi : Inport
  Theta : Inport  Port=2
  Psi : Inport  Port=3
  Product : Product  Inputs=3  Multiplication=Matrix(*)
  R1 : Subsystem
  R3_1 : Subsystem
  R3_2 : Subsystem
  A : Outport
  wires:
  R3_2/1(R3) -> Product/1
  R1/1(R1) -> Product/2
  R3_1/1(R3) -> Product/3
  Phi/1 -> R3_1/1(x)
  Theta/1 -> R1/1(x)
  Psi/1 -> R3_2/1(x)
  Product/1 -> A/1

== system sat_dist_sim/Attitude Euler Angles/Subsystem1/If Action Subsystem1/Kin 312/Euler Angles ==
  omega : Inport
  Constant : Constant  Value=s0
  Demux : Demux  Outputs=3
  phi : Subsystem
  psi : Subsystem
  th : Subsystem
  Phi : Outport
  Theta : Outport  Port=2
  Psi : Outport  Port=3
  wires:
  th/1(theta) -> Theta/1, psi/2(Th), phi/2(th)
  psi/1(psi) -> phi/3(psi), th/2(psi), psi/3(psi_), Psi/1
  phi/1(phi) -> Phi/1
  omega/1 -> psi/1(omega), phi/1(omega), th/1(omega)
  Demux/3 -> phi/4(In4)
  Demux/2 -> th/3(In3)
  Demux/1 -> psi/4(In4)
  Constant/1 -> Demux/1

== system sat_dist_sim/Attitude Euler Angles/Subsystem1/If Action Subsystem1/Kin 312/Subsystem ==
  phi : Inport
  theta : Inport  Port=2
  psi : Inport  Port=3
  Product : Product  Inputs=3  Multiplication=Matrix(*)
  R1 : Subsystem
  R2 : Subsystem
  R3 : Subsystem
  A : Outport
  wires:
  R1/1(R1) -> Product/2
  R3/1(R3) -> Product/3
  R2/1(R2) -> Product/1
  phi/1 -> R3/1(x)
  theta/1 -> R1/1(x)
  psi/1 -> R2/1(x)
  Product/1 -> A/1

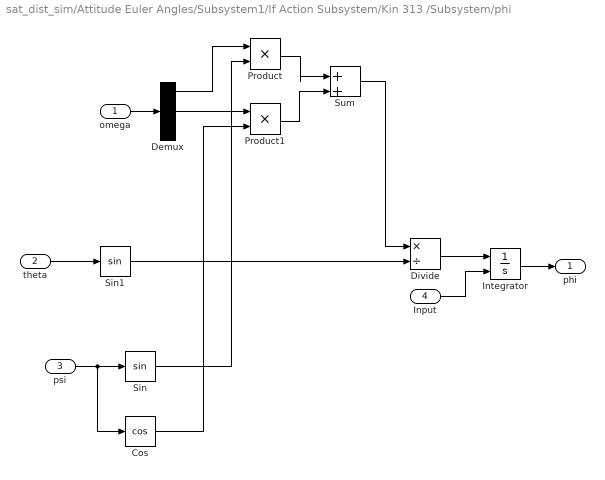
== system sat_dist_sim/Attitude Euler Angles/Subsystem1/If Action Subsystem/Kin 313 /Subsystem/phi ==
  omega : Inport
  theta : Inport  Port=2
  psi : Inport  Port=3
  Input : Inport  Port=4
  Cos : Trigonometry  Operator=cos
  Demux : Demux  Outputs=3
  Divide : Product  Inputs=*/
  Integrator : Integrator  InitialConditionSource=external  WrappedStateUpperValue=2*pi  WrappedStateLowerValue=0
  Product : Product
  Product1 : Product
  Sin : Trigonometry
  Sin1 : Trigonometry
  Sum : Sum  Inputs=|++
  phi : Outport
  wires:
  omega/1 -> Demux/1
  Demux/1 -> Product/1
  psi/1 -> Cos/1, Sin/1
  Sin/1 -> Product/2
  Demux/2 -> Product1/1
  Cos/1 -> Product1/2
  Product/1 -> Sum/1
  Product1/1 -> Sum/2
  theta/1 -> Sin1/1
  Sum/1 -> Divide/1
  Sin1/1 -> Divide/2
  Divide/1 -> Integrator/1
  Integrator/1 -> phi/1
  Input/1 -> Integrator/2

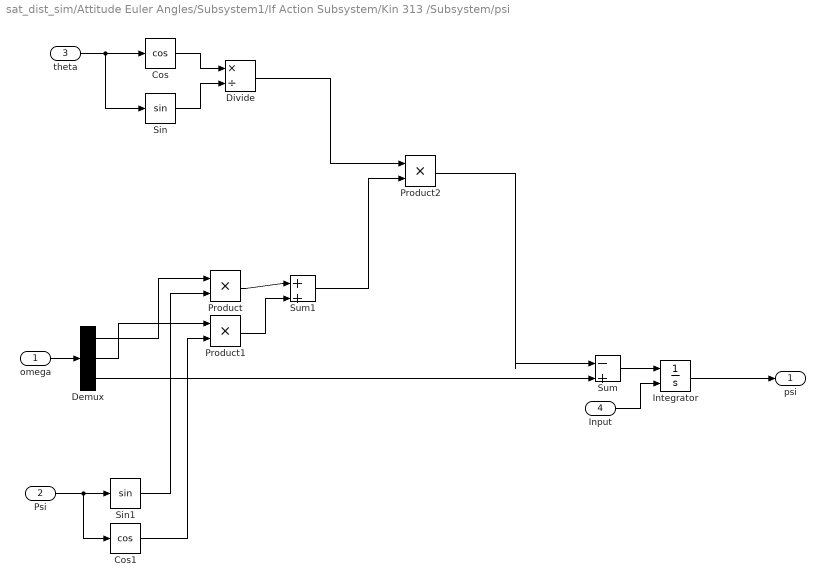
== system sat_dist_sim/Attitude Euler Angles/Subsystem1/If Action Subsystem/Kin 313 /Subsystem/psi ==
  omega : Inport
  Psi : Inport  Port=2
  theta : Inport  Port=3
  Input : Inport  Port=4
  Cos : Trigonometry  Operator=cos
  Cos1 : Trigonometry  Operator=cos
  Demux : Demux  Outputs=3
  Divide : Product  Inputs=*/
  Integrator : Integrator  InitialConditionSource=external  WrappedStateUpperValue=2*pi  WrappedStateLowerValue=0
  Product : Product
  Product1 : Product
  Product2 : Product
  Sin : Trigonometry
  Sin1 : Trigonometry
  Sum : Sum  Inputs=|-+
  Sum1 : Sum  Inputs=|++
  psi : Outport
  wires:
  omega/1 -> Demux/1
  theta/1 -> Sin/1, Cos/1
  Cos/1 -> Divide/1
  Sin/1 -> Divide/2
  Psi/1 -> Sin1/1, Cos1/1
  Demux/1 -> Product/1
  Sin1/1 -> Product/2
  Demux/2 -> Product1/1
  Cos1/1 -> Product1/2
  Product/1 -> Sum1/1
  Product1/1 -> Sum1/2
  Divide/1 -> Product2/1
  Sum1/1 -> Product2/2
  Demux/3 -> Sum/2
  Product2/1 -> Sum/1
  Sum/1 -> Integrator/1
  Integrator/1 -> psi/1
  Input/1 -> Integrator/2

== system sat_dist_sim/Attitude Euler Angles/Subsystem1/If Action Subsystem/Kin 313 /Subsystem/theta ==
  omega : Inport
  psi : Inport  Port=2
  Input : Inport  Port=3
  Cos : Trigonometry  Operator=cos
  Demux : Demux  Outputs=3
  Integrator : Integrator  InitialConditionSource=external  WrappedStateUpperValue=2*pi  WrappedStateLowerValue=0
  Product : Product
  Product1 : Product
  Sin : Trigonometry
  Sum : Sum  Inputs=|++
  theta : Outport
  wires:
  omega/1 -> Demux/1
  psi/1 -> Cos/1, Sin/1
  Demux/1 -> Product/1
  Sin/1 -> Product/2
  Demux/2 -> Product1/1
  Cos/1 -> Product1/2
  Product/1 -> Sum/1
  Product1/1 -> Sum/2
  Sum/1 -> Integrator/1
  Integrator/1 -> theta/1
  Input/1 -> Integrator/2

== system sat_dist_sim/Attitude Euler Angles/Subsystem1/If Action Subsystem/Kin 313 /Subsystem1/R1 ==
  x : Inport
  Constant : Constant  Value=[1; 0; 0]
  Constant1 : Constant  Value=0
  Cos : Trigonometry  Operator=cos
  Gain : Gain  Gain=-1
  Matrix Concatenate : Concatenate  NumInputs=3  Mode=Multidimensional array  ConcatenateDimension=2
  Sin : Trigonometry
  Vector Concatenate : Concatenate  NumInputs=3
  Vector Concatenate1 : Concatenate  NumInputs=3
  R1 : Outport
  wires:
  Sin/1 -> Gain/1, Vector Concatenate/2
  Gain/1 -> Vector Concatenate1/3
  Cos/1 -> Vector Concatenate1/2, Vector Concatenate/3
  Constant1/1 -> Vector Concatenate1/1, Vector Concatenate/1
  Vector Concatenate/1 -> Matrix Concatenate/3
  Constant/1 -> Matrix Concatenate/1
  Vector Concatenate1/1 -> Matrix Concatenate/2
  x/1 -> Sin/1, Cos/1
  Matrix Concatenate/1 -> R1/1

== system sat_dist_sim/Attitude Euler Angles/Subsystem1/If Action Subsystem/Kin 313 /Subsystem1/R3_1 ==
  x : Inport
  Constant : Constant  Value=[0; 0; 1]
  Constant1 : Constant  Value=0
  Cos : Trigonometry  Operator=cos
  Gain : Gain  Gain=-1
  Matrix Concatenate : Concatenate  NumInputs=3  Mode=Multidimensional array  ConcatenateDimension=2
  Sin : Trigonometry
  Vector Concatenate : Concatenate  NumInputs=3
  Vector Concatenate1 : Concatenate  NumInputs=3
  R3 : Outport
  wires:
  Matrix Concatenate/1 -> R3/1
  Constant1/1 -> Vector Concatenate1/3, Vector Concatenate/3
  x/1 -> Cos/1, Sin/1
  Vector Concatenate1/1 -> Matrix Concatenate/2
  Gain/1 -> Vector Concatenate/2
  Constant/1 -> Matrix Concatenate/3
  Cos/1 -> Vector Concatenate/1, Vector Concatenate1/2
  Sin/1 -> Gain/1, Vector Concatenate1/1
  Vector Concatenate/1 -> Matrix Concatenate/1

== system sat_dist_sim/Attitude Euler Angles/Subsystem1/If Action Subsystem/Kin 313 /Subsystem1/R3_2 ==
  x : Inport
  Constant : Constant  Value=[0; 0; 1]
  Constant1 : Constant  Value=0
  Cos : Trigonometry  Operator=cos
  Gain : Gain  Gain=-1
  Matrix Concatenate : Concatenate  NumInputs=3  Mode=Multidimensional array  ConcatenateDimension=2
  Sin : Trigonometry
  Vector Concatenate : Concatenate  NumInputs=3
  Vector Concatenate1 : Concatenate  NumInputs=3
  R3 : Outport
  wires:
  Vector Concatenate/1 -> Matrix Concatenate/1
  Sin/1 -> Vector Concatenate1/1, Gain/1
  Cos/1 -> Vector Concatenate1/2, Vector Concatenate/1
  Constant/1 -> Matrix Concatenate/3
  Gain/1 -> Vector Concatenate/2
  Vector Concatenate1/1 -> Matrix Concatenate/2
  x/1 -> Sin/1, Cos/1
  Constant1/1 -> Vector Concatenate/3, Vector Concatenate1/3
  Matrix Concatenate/1 -> R3/1

== system sat_dist_sim/Attitude Euler Angles/Subsystem1/If Action Subsystem1/Kin 312/Euler Angles/phi ==
  omega : Inport
  th : Inport  Port=2
  psi : Inport  Port=3
  In4 : Inport  Port=4
  Cos : Trigonometry  Operator=cos
  Cos1 : Trigonometry  Operator=cos
  Demux : Demux  Outputs=3
  Divide : Product  Inputs=*/
  Integrator : Integrator  InitialConditionSource=external  InitialCondition=phi0  WrappedStateUpperValue=2*pi  WrappedStateLowerValue=0
  Product : Product
  Product1 : Product
  Sin : Trigonometry
  Sum : Sum  Inputs=|-+
  phi : Outport
  wires:
  omega/1 -> Demux/1
  psi/1 -> Cos/1, Sin/1
  Demux/1 -> Product/1
  Sin/1 -> Product/2
  Demux/3 -> Product1/1
  Cos/1 -> Product1/2
  Product/1 -> Sum/1
  Product1/1 -> Sum/2
  th/1 -> Cos1/1
  Sum/1 -> Divide/1
  Cos1/1 -> Divide/2
  Divide/1 -> Integrator/1
  Integrator/1 -> phi/1
  In4/1 -> Integrator/2

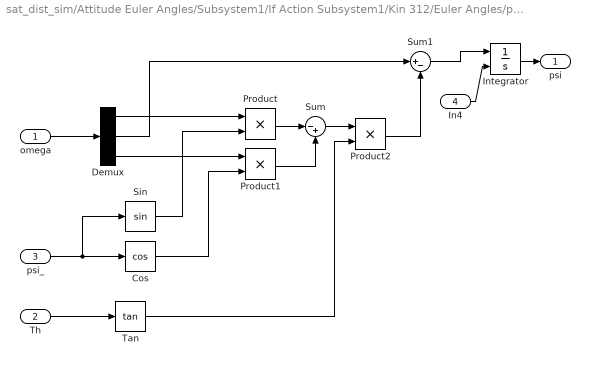
== system sat_dist_sim/Attitude Euler Angles/Subsystem1/If Action Subsystem1/Kin 312/Euler Angles/psi ==
  omega : Inport
  Th : Inport  Port=2
  psi_ : Inport  Port=3
  In4 : Inport  Port=4
  Cos : Trigonometry  Operator=cos
  Demux : Demux  Outputs=3
  Integrator : Integrator  InitialConditionSource=external  InitialCondition=psi0  WrappedStateUpperValue=2*pi  WrappedStateLowerValue=0
  Product : Product
  Product1 : Product
  Product2 : Product
  Sin : Trigonometry
  Sum : Sum  Inputs=|-+
  Sum1 : Sum  Inputs=|+-
  Tan : Trigonometry  Operator=tan
  psi : Outport
  wires:
  omega/1 -> Demux/1
  psi_/1 -> Sin/1, Cos/1
  Demux/1 -> Product/1
  Sin/1 -> Product/2
  Demux/3 -> Product1/1
  Cos/1 -> Product1/2
  Th/1 -> Tan/1
  Product/1 -> Sum/1
  Product1/1 -> Sum/2
  Sum/1 -> Product2/1
  Tan/1 -> Product2/2
  Product2/1 -> Sum1/2
  Demux/2 -> Sum1/1
  Sum1/1 -> Integrator/1
  Integrator/1 -> psi/1
  In4/1 -> Integrator/2

== system sat_dist_sim/Attitude Euler Angles/Subsystem1/If Action Subsystem1/Kin 312/Euler Angles/th ==
  omega : Inport
  psi : Inport  Port=2
  In3 : Inport  Port=3
  Cos : Trigonometry  Operator=cos
  Demux : Demux  Outputs=3
  Integrator : Integrator  InitialConditionSource=external  InitialCondition=theta0  WrappedStateUpperValue=2*pi  WrappedStateLowerValue=0
  Product : Product
  Product1 : Product
  Sin : Trigonometry
  Sum : Sum  Inputs=|++
  theta : Outport
  wires:
  omega/1 -> Demux/1
  psi/1 -> Sin/1, Cos/1
  Demux/1 -> Product/1
  Cos/1 -> Product/2
  Demux/3 -> Product1/1
  Sin/1 -> Product1/2
  Product/1 -> Sum/1
  Product1/1 -> Sum/2
  Sum/1 -> Integrator/1
  Integrator/1 -> theta/1
  In3/1 -> Integrator/2

== system sat_dist_sim/Attitude Euler Angles/Subsystem1/If Action Subsystem1/Kin 312/Subsystem/R1 ==
  x : Inport
  Constant : Constant  Value=[1; 0; 0]
  Constant1 : Constant  Value=0
  Cos : Trigonometry  Operator=cos
  Gain : Gain  Gain=-1
  Matrix Concatenate : Concatenate  NumInputs=3  Mode=Multidimensional array  ConcatenateDimension=2
  Sin : Trigonometry
  Vector Concatenate : Concatenate  NumInputs=3
  Vector Concatenate1 : Concatenate  NumInputs=3
  R1 : Outport
  wires:
  Matrix Concatenate/1 -> R1/1
  x/1 -> Cos/1, Sin/1
  Vector Concatenate1/1 -> Matrix Concatenate/2
  Constant/1 -> Matrix Concatenate/1
  Vector Concatenate/1 -> Matrix Concatenate/3
  Constant1/1 -> Vector Concatenate/1, Vector Concatenate1/1
  Cos/1 -> Vector Concatenate/3, Vector Concatenate1/2
  Gain/1 -> Vector Concatenate1/3
  Sin/1 -> Vector Concatenate/2, Gain/1

== system sat_dist_sim/Attitude Euler Angles/Subsystem1/If Action Subsystem1/Kin 312/Subsystem/R2 ==
  x : Inport
  Constant : Constant  Value=[0; 1; 0]
  Constant1 : Constant  Value=0
  Cos : Trigonometry  Operator=cos
  Gain : Gain  Gain=-1
  Matrix Concatenate : Concatenate  NumInputs=3  Mode=Multidimensional array  ConcatenateDimension=2
  Sin : Trigonometry
  Vector Concatenate : Concatenate  NumInputs=3
  Vector Concatenate1 : Concatenate  NumInputs=3
  R2 : Outport
  wires:
  Vector Concatenate/1 -> Matrix Concatenate/1
  x/1 -> Sin/1, Cos/1
  Matrix Concatenate/1 -> R2/1
  Constant/1 -> Matrix Concatenate/2
  Vector Concatenate1/1 -> Matrix Concatenate/3
  Constant1/1 -> Vector Concatenate/2, Vector Concatenate1/2
  Cos/1 -> Vector Concatenate1/3, Vector Concatenate/1
  Sin/1 -> Gain/1, Vector Concatenate/3
  Gain/1 -> Vector Concatenate1/1

== system sat_dist_sim/Attitude Euler Angles/Subsystem1/If Action Subsystem1/Kin 312/Subsystem/R3 ==
  x : Inport
  Constant : Constant  Value=[0; 0; 1]
  Constant1 : Constant  Value=0
  Cos : Trigonometry  Operator=cos
  Gain : Gain  Gain=-1
  Matrix Concatenate : Concatenate  NumInputs=3  Mode=Multidimensional array  ConcatenateDimension=2
  Sin : Trigonometry
  Vector Concatenate : Concatenate  NumInputs=3
  Vector Concatenate1 : Concatenate  NumInputs=3
  R3 : Outport
  wires:
  Vector Concatenate/1 -> Matrix Concatenate/1
  Sin/1 -> Vector Concatenate1/1, Gain/1
  Cos/1 -> Vector Concatenate1/2, Vector Concatenate/1
  Constant/1 -> Matrix Concatenate/3
  Gain/1 -> Vector Concatenate/2
  Vector Concatenate1/1 -> Matrix Concatenate/2
  x/1 -> Sin/1, Cos/1
  Constant1/1 -> Vector Concatenate/3, Vector Concatenate1/3
  Matrix Concatenate/1 -> R3/1
